simulink model "Shanthan_Heeirthan_EE469S3D_R45 (1)"  (R2023a)
settings: Solver=FixedStepDiscrete  StartTime=0.0  StopTime=120  FixedStep=dt0  RelTol=1e-3  EnableMultiTasking=on
PostLoadFcn:
  | %Set the size for the model
  | set_param(gcs,'Location',[10 10 1270 970])
  | %Set the zoom factor for the model
  | set_param(gcs,'ZoomFactor','100')
InitFcn:
  | tic
  | % Students Add call to their M-file HERE
  | Shanthan_Heeirthan_EE460_Final
  | INIT_S3D_01
StartFcn:
  | tend0=toc;
  | tic;
StopFcn:
  | tend=toc;
  | disp(['Simulation time = ' num2str(tout(end)) ' sec'])
  | disp(['Real time = ' num2str(tend) ' sec'])
  | title('DONE')
  | SCORE=round((max(0,120-tout(end)-tend0))*4+10*(40-FuelBurned)+sum(100*double(PDONE)-100*double(PDONE<.5)));
  | PlotS3D(PlotInput);
  | text(15,22,['S: ' num2str(SCORE)]);
values from neighbouring files (symbols this model uses):
  A = [0 1 0 0 0 0 ... (first row only)    [Shanthan_Heeirthan_EE460_Final (1).m]
  B = [0 0 0 ... (first row only)    [Shanthan_Heeirthan_EE460_Final (1).m]
  bm = [1 1 -1 -1 0 0 0 0; 0 0 0 0 -1 1 1 -1; -1 1 -1 1 3 -3 3 -3]    [Shanthan_Heeirthan_EE460_Final (1).m]
  C = [1 0 0 0 0 0 ... (first row only)    [Shanthan_Heeirthan_EE460_Final (1).m]
  D = [0 0 0 ... (first row only)    [Shanthan_Heeirthan_EE460_Final (1).m]
  Denchptheta = TFchptheta.Den{1}    [Shanthan_Heeirthan_EE460_Final (1).m]
  Denchpxy = TFchpxy.Den{1}    [Shanthan_Heeirthan_EE460_Final (1).m]
  Denclptheta = TFclptheta.Den{1}    [Shanthan_Heeirthan_EE460_Final (1).m]
  Denclpxy = TFclpxy.Den{1}    [Shanthan_Heeirthan_EE460_Final (1).m]
  Denlp = TFlp.Den{1}    [Shanthan_Heeirthan_EE460_Final (1).m]
  Kd = 2.1+0    (= 2.1)    [Shanthan_Heeirthan_EE460_Final (1).m]
  Ki = 0.0001    [Shanthan_Heeirthan_EE460_Final (1).m]
  Kp = 1.1+0.2    (= 1.3)    [Shanthan_Heeirthan_EE460_Final (1).m]
  L = place(A',C',ep)'    [Shanthan_Heeirthan_EE460_Final (1).m]
  Numchptheta = TFchptheta.Num{1}    [Shanthan_Heeirthan_EE460_Final (1).m]
  Numchpxy = TFchpxy.Num{1}    [Shanthan_Heeirthan_EE460_Final (1).m]
  Numclptheta = TFclptheta.Num{1}    [Shanthan_Heeirthan_EE460_Final (1).m]
  Numclpxy = TFclpxy.Num{1}    [Shanthan_Heeirthan_EE460_Final (1).m]
  Numlp = TFlp.Num{1}    [Shanthan_Heeirthan_EE460_Final (1).m]
  Pnewdata = [LVL.P1 LVL.P2 LVL.P3 LVL.P4]    [Shanthan_Heeirthan_EE460_Final (1).m]
  Sconfig = 1    [Shanthan_Heeirthan_EE460_Final (1).m]
  TFP1 = 2    [Shanthan_Heeirthan_EE460_Final (1).m]
  TFP1z = 1    [Shanthan_Heeirthan_EE460_Final (1).m]
  TFP2 = 2    [Shanthan_Heeirthan_EE460_Final (1).m]
  TFP2z = 1    [Shanthan_Heeirthan_EE460_Final (1).m]
  TFP3 = 2    [Shanthan_Heeirthan_EE460_Final (1).m]
  TFP3z = 1    [Shanthan_Heeirthan_EE460_Final (1).m]
  TFP4 = 2    [Shanthan_Heeirthan_EE460_Final (1).m]
  TFP4z = 1    [Shanthan_Heeirthan_EE460_Final (1).m]
  wcf = 2    [Shanthan_Heeirthan_EE460_Final (1).m]
  wcft = 10    [Shanthan_Heeirthan_EE460_Final (1).m]
undefined symbols (not defined in the file or in its folder): d2r, DiscIntNeverNeededParam, dt, dt0, fr, HM_S, HM_U, J, Jbase, JC0, L13, L24, LVL, M, M1, M2, M3, M4, mdti, Pdata, PTvec, r2d, SLIM, SQ, SSF, TOLdata, ULIM
libraries: simulink x85, aerolibanimutils x1, matrix_library x1
(part 6 of 7)

== system Shanthan_Heeirthan_EE469S3D_R45 (1)/control_law/CMD/CMDprocess/CommandTypes/Ramp1 ==
  ICCMDs : Inport
  Action Port : ActionPort  ActionPortLabel=if(u1 < 1.5)
  Bus Creator : BusCreator  Inputs=2
  Bus Selector : BusSelector  OutputSignals=X_CMD,Y_CMD
  Bus Selector1 : BusSelector  OutputSignals=CMDS.XdesCMD,CMDS.YdesCMD  OutputAsBus=on
  Gain : Gain
  Gain1 : Gain
  Gain2 : Gain
  Mux : Mux  Inputs=3
  Xcmd1 : Subsystem
  Ycmd : Subsystem
  Zcmd : Subsystem
  RMP_CMDS : Outport
  wires:
  Zcmd/1(ZCMD) -> Gain2/1
  Xcmd1/1(XCMD) -> Bus Creator/1
  Ycmd/1(XCMD) -> Bus Creator/2
  Mux/1 -> RMP_CMDS/1  "RMP_CMDS"
  Bus Creator/1 -> Bus Selector/1
  Bus Selector/2 -> Gain1/1  "<Y_CMD>"
  Bus Selector/1 -> Gain/1  "<X_CMD>"
  Gain/1 -> Mux/1
  Gain1/1 -> Mux/2
  ICCMDs/1 -> Bus Selector1/1, Zcmd/1(Sensed), Ycmd/1(ICCMDs), Xcmd1/1(ICCMDst)
  Bus Selector1/1 -> Zcmd/2(CMDS)  "CMDS"
  Gain2/1 -> Mux/3

== system Shanthan_Heeirthan_EE469S3D_R45 (1)/control_law/CMD/CMDprocess/CommandTypes/Ramp2 ==
  ICCMDs : Inport
  Action Port : ActionPort  ActionPortLabel=elseif( u1<3.5)
  Bus Creator : BusCreator  Inputs=2
  Bus Selector : BusSelector  OutputSignals=X_CMD,Y_CMD
  Bus Selector1 : BusSelector  OutputSignals=CMDS.XdesCMD,CMDS.YdesCMD  OutputAsBus=on
  Gain : Gain
  Gain1 : Gain
  Gain2 : Gain
  Mux : Mux  Inputs=3
  Xcmd1 : Subsystem
  Ycmd : Subsystem
  Zcmd : Subsystem
  RMP_CMDS : Outport
  wires:
  Zcmd/1(ZCMD) -> Gain2/1
  Xcmd1/1(XCMD) -> Bus Creator/1
  Ycmd/1(XCMD) -> Bus Creator/2
  Mux/1 -> RMP_CMDS/1  "RMP_CMDS"
  Bus Creator/1 -> Bus Selector/1
  Bus Selector/2 -> Gain1/1  "<Y_CMD>"
  Bus Selector/1 -> Gain/1  "<X_CMD>"
  Gain/1 -> Mux/1
  Gain1/1 -> Mux/2
  ICCMDs/1 -> Bus Selector1/1, Zcmd/1(Sensed), Ycmd/1(ICCMDs), Xcmd1/1(ICCMDst)
  Bus Selector1/1 -> Zcmd/2(CMDS)  "CMDS"
  Gain2/1 -> Mux/3

== system Shanthan_Heeirthan_EE469S3D_R45 (1)/control_law/CMD/CMDprocess/CommandTypes/Ramp3 ==
  ICCMDs : Inport
  Action Port : ActionPort  ActionPortLabel=else
  Bus Creator : BusCreator  Inputs=2
  Bus Selector : BusSelector  OutputSignals=X_CMD,Y_CMD
  Bus Selector1 : BusSelector  OutputSignals=CMDS.XdesCMD,CMDS.YdesCMD  OutputAsBus=on
  Gain : Gain
  Gain1 : Gain
  Gain2 : Gain
  Mux : Mux  Inputs=3
  Xcmd1 : Subsystem
  Ycmd : Subsystem
  Zcmd : Subsystem
  RMP_CMDS : Outport
  wires:
  Zcmd/1(ZCMD) -> Gain2/1
  Xcmd1/1(XCMD) -> Bus Creator/1
  Ycmd/1(XCMD) -> Bus Creator/2
  Mux/1 -> RMP_CMDS/1  "RMP_CMDS"
  Bus Creator/1 -> Bus Selector/1
  Bus Selector/2 -> Gain1/1  "<Y_CMD>"
  Bus Selector/1 -> Gain/1  "<X_CMD>"
  Gain/1 -> Mux/1
  Gain1/1 -> Mux/2
  ICCMDs/1 -> Bus Selector1/1, Zcmd/1(Sensed), Ycmd/1(ICCMDs), Xcmd1/1(ICCMDst)
  Bus Selector1/1 -> Zcmd/2(CMDS)  "CMDS"
  Gain2/1 -> Mux/3

== system Shanthan_Heeirthan_EE469S3D_R45 (1)/control_law/CMD/CMDprocess/CommandTypes/Ramp4 ==
  ICCMDs : Inport
  Action Port : ActionPort  ActionPortLabel=elseif(u1<2.5)
  Bus Creator : BusCreator  Inputs=2
  Bus Selector : BusSelector  OutputSignals=X_CMD,Y_CMD
  Bus Selector1 : BusSelector  OutputSignals=CMDS.XdesCMD,CMDS.YdesCMD  OutputAsBus=on
  Gain : Gain
  Gain1 : Gain
  Gain2 : Gain
  Mux : Mux  Inputs=3
  Xcmd1 : Subsystem
  Ycmd : Subsystem
  Zcmd : Subsystem
  RMP_CMDS : Outport
  wires:
  Zcmd/1(ZCMD) -> Gain2/1
  Xcmd1/1(XCMD) -> Bus Creator/1
  Ycmd/1(YCMD) -> Bus Creator/2
  Mux/1 -> RMP_CMDS/1  "RMP_CMDS"
  Bus Creator/1 -> Bus Selector/1
  Bus Selector/2 -> Gain1/1  "<Y_CMD>"
  Bus Selector/1 -> Gain/1  "<X_CMD>"
  Gain/1 -> Mux/1
  Gain1/1 -> Mux/2
  ICCMDs/1 -> Bus Selector1/1, Zcmd/1(Sensed), Ycmd/1(ICCMDs), Xcmd1/1(ICCMDst)
  Bus Selector1/1 -> Zcmd/2(CMDS)  "CMDS"
  Gain2/1 -> Mux/3

== system Shanthan_Heeirthan_EE469S3D_R45 (1)/control_law/CMD/CMDprocess/CommandTypes/Ramp1/Xcmd1 ==
  ICCMDst : Inport
  Bus Selector : BusSelector  OutputSignals=ICs.ICX,CMDS.XdesCMD
  Constant : Constant  Value=TFP1
  Gain : Gain  Gain=1/TFP1
  Gain1 : Gain
  Product : Product
  Sum : Sum  Inputs=|++
  Sum1 : Sum  Inputs=|-+
  VariableTimer : Subsystem
  XCMD : Outport
  wires:
  Gain1/1 -> XCMD/1  "X_CMD"
  Sum/1 -> Gain1/1  "qc"
  Bus Selector/2 -> Sum1/2  "<XdesCMD>"
  Bus Selector/1 -> Sum/1, Sum1/1  "<ICX>"
  ICCMDst/1 -> Bus Selector/1
  Constant/1 -> VariableTimer/1(TFramp)  "TFRamp"
  Product/1 -> Sum/2  "qcdot"
  Sum1/1 -> Gain/1
  VariableTimer/1(Time_sec) -> Product/2
  Gain/1 -> Product/1

== system Shanthan_Heeirthan_EE469S3D_R45 (1)/control_law/CMD/CMDprocess/CommandTypes/Ramp1/Ycmd ==
  ICCMDs : Inport
  Bus Selector : BusSelector  OutputSignals=ICs.ICY,CMDS.YdesCMD
  Constant : Constant  Value=TFP1
  Gain : Gain  Gain=1/TFP1
  Gain1 : Gain
  Product : Product
  Sum : Sum  Inputs=|++
  Sum1 : Sum  Inputs=|-+
  VariableTimer : Subsystem
  XCMD : Outport
  wires:
  VariableTimer/1(Time_sec) -> Product/2
  Product/1 -> Sum/2  "qcdot"
  Bus Selector/1 -> Sum/1, Sum1/1  "<ICY>"
  Gain1/1 -> XCMD/1  "Y_CMD"
  Sum/1 -> Gain1/1  "qc"
  Sum1/1 -> Gain/1
  Constant/1 -> VariableTimer/1(TFramp)  "TFRamp"
  ICCMDs/1 -> Bus Selector/1
  Bus Selector/2 -> Sum1/2  "<YdesCMD>"
  Gain/1 -> Product/1

== system Shanthan_Heeirthan_EE469S3D_R45 (1)/control_law/CMD/CMDprocess/CommandTypes/Ramp1/Zcmd ==
  Sensed : Inport
  CMDS : Inport  Port=2
  Bus Selector : BusSelector  OutputSignals=ICs.ICZ,CMDS.ZdesCMD
  Bus Selector2 : BusSelector  OutputSignals=Sensed.X1_m,Sensed.Y_m  OutputAsBus=on
  Constant : Constant  Value=0
  Data Type Conversion1 : DataTypeConversion  OutDataTypeStr=boolean  SaturateOnIntegerOverflow=off  RndMeth=Floor
  Gain : Gain  Gain=1/TFP1z
  If : If  IfExpression=u1 == 0
  Merge : Merge
  Product : Product
  StartTimer : Subsystem  TreatAsAtomicUnit=on
  Subsystem : Subsystem
  Sum : Sum  Inputs=|++
  Sum1 : Sum  Inputs=|-+
  Switch : Switch  Criteria=u2 > Threshold  SaturateOnIntegerOverflow=off  InputSameDT=off
  Terminator : Terminator
  ZCMD : Outport
  wires:
  Sum/1 -> ZCMD/1  "qc"
  Bus Selector/2 -> Sum1/2  "<ZdesCMD>"
  Gain/1 -> Product/1
  Bus Selector/1 -> Sum/1, Sum1/1  "<ICZ>"
  Sensed/1 -> Bus Selector2/1, Bus Selector/1
  Product/1 -> Sum/2  "qcdot"
  Sum1/1 -> Gain/1
  Switch/1 -> Product/2
  StartTimer/1(Out1) -> Switch/3
  Merge/1 -> Data Type Conversion1/1
  Data Type Conversion1/1 -> Switch/2, If/1
  Subsystem/1(Iftrue) -> Switch/1
  Subsystem/3(Toggle2) -> Merge/2
  CMDS/1 -> Subsystem/2(CMDS)  "CMDS"
  If/1 -> StartTimer/Action
  Bus Selector2/1 -> Subsystem/1(Sensed)  "Sensed"
  Subsystem/2(Toggle1) -> Merge/1
  Constant/1 -> Subsystem/3(Pmodeinit)  "Pmodeinit"
  If/2 -> Terminator/1

== system Shanthan_Heeirthan_EE469S3D_R45 (1)/control_law/CMD/CMDprocess/CommandTypes/Ramp2/Xcmd1 ==
  ICCMDst : Inport
  Bus Selector : BusSelector  OutputSignals=ICs.ICX,CMDS.XdesCMD
  Constant : Constant  Value=TFP3
  Gain : Gain  Gain=1/TFP3
  Gain1 : Gain
  Product : Product
  Sum : Sum  Inputs=|++
  Sum1 : Sum  Inputs=|-+
  VariableTimer : Subsystem
  XCMD : Outport
  wires:
  Gain1/1 -> XCMD/1  "X_CMD"
  Sum/1 -> Gain1/1  "qc"
  Bus Selector/2 -> Sum1/2  "<XdesCMD>"
  Bus Selector/1 -> Sum/1, Sum1/1  "<ICX>"
  ICCMDst/1 -> Bus Selector/1
  Constant/1 -> VariableTimer/1(TFramp)  "TFRamp"
  Product/1 -> Sum/2  "qcdot"
  Sum1/1 -> Gain/1
  VariableTimer/1(Time_sec) -> Product/2
  Gain/1 -> Product/1

== system Shanthan_Heeirthan_EE469S3D_R45 (1)/control_law/CMD/CMDprocess/CommandTypes/Ramp2/Ycmd ==
  ICCMDs : Inport
  Bus Selector : BusSelector  OutputSignals=ICs.ICY,CMDS.YdesCMD
  Constant : Constant  Value=TFP3
  Gain : Gain  Gain=1/TFP3
  Gain1 : Gain
  Product : Product
  Sum : Sum  Inputs=|++
  Sum1 : Sum  Inputs=|-+
  VariableTimer : Subsystem
  XCMD : Outport
  wires:
  VariableTimer/1(Time_sec) -> Product/2
  Product/1 -> Sum/2  "qcdot"
  Bus Selector/1 -> Sum/1, Sum1/1  "<ICY>"
  Gain1/1 -> XCMD/1  "Y_CMD"
  Sum/1 -> Gain1/1  "qc"
  Sum1/1 -> Gain/1
  Constant/1 -> VariableTimer/1(TFramp)  "TFRamp"
  ICCMDs/1 -> Bus Selector/1
  Bus Selector/2 -> Sum1/2  "<YdesCMD>"
  Gain/1 -> Product/1

== system Shanthan_Heeirthan_EE469S3D_R45 (1)/control_law/CMD/CMDprocess/CommandTypes/Ramp2/Zcmd ==
  Sensed : Inport
  CMDS : Inport  Port=2
  Bus Selector : BusSelector  OutputSignals=ICs.ICZ,CMDS.ZdesCMD
  Bus Selector2 : BusSelector  OutputSignals=Sensed.X1_m,Sensed.Y_m  OutputAsBus=on
  Constant : Constant  Value=0
  Data Type Conversion1 : DataTypeConversion  OutDataTypeStr=boolean  SaturateOnIntegerOverflow=off  RndMeth=Floor
  Gain : Gain  Gain=1/TFP3z
  If : If  IfExpression=u1 == 0
  Merge : Merge
  Product : Product
  StartTimer : Subsystem  TreatAsAtomicUnit=on
  Subsystem : Subsystem
  Sum : Sum  Inputs=|++
  Sum1 : Sum  Inputs=|-+
  Switch : Switch  Criteria=u2 > Threshold  SaturateOnIntegerOverflow=off  InputSameDT=off
  Terminator : Terminator
  ZCMD : Outport
  wires:
  Sum/1 -> ZCMD/1  "qc"
  Bus Selector/2 -> Sum1/2  "<ZdesCMD>"
  Gain/1 -> Product/1
  Bus Selector/1 -> Sum/1, Sum1/1  "<ICZ>"
  Sensed/1 -> Bus Selector2/1, Bus Selector/1
  Product/1 -> Sum/2  "qcdot"
  Sum1/1 -> Gain/1
  Switch/1 -> Product/2
  StartTimer/1(Out1) -> Switch/3
  Merge/1 -> Data Type Conversion1/1
  Data Type Conversion1/1 -> Switch/2, If/1
  Subsystem/1(Iftrue) -> Switch/1
  Subsystem/3(Toggle2) -> Merge/2
  CMDS/1 -> Subsystem/2(CMDS)  "CMDS"
  If/1 -> StartTimer/Action
  Bus Selector2/1 -> Subsystem/1(Sensed)  "Sensed"
  Subsystem/2(Toggle1) -> Merge/1
  Constant/1 -> Subsystem/3(Pmodeinit)  "Pmodeinit"
  If/2 -> Terminator/1

== system Shanthan_Heeirthan_EE469S3D_R45 (1)/control_law/CMD/CMDprocess/CommandTypes/Ramp3/Xcmd1 ==
  ICCMDst : Inport
  Bus Selector : BusSelector  OutputSignals=ICs.ICX,CMDS.XdesCMD
  Constant : Constant  Value=TFP4
  Gain : Gain  Gain=1/TFP4
  Gain1 : Gain
  Product : Product
  Sum : Sum  Inputs=|++
  Sum1 : Sum  Inputs=|-+
  VariableTimer : Subsystem
  XCMD : Outport
  wires:
  Gain1/1 -> XCMD/1  "X_CMD"
  Sum/1 -> Gain1/1  "qc"
  Bus Selector/2 -> Sum1/2  "<XdesCMD>"
  Bus Selector/1 -> Sum/1, Sum1/1  "<ICX>"
  ICCMDst/1 -> Bus Selector/1
  Constant/1 -> VariableTimer/1(TFramp)  "TFRamp"
  Product/1 -> Sum/2  "qcdot"
  Sum1/1 -> Gain/1
  VariableTimer/1(Time_sec) -> Product/2
  Gain/1 -> Product/1

== system Shanthan_Heeirthan_EE469S3D_R45 (1)/control_law/CMD/CMDprocess/CommandTypes/Ramp3/Ycmd ==
  ICCMDs : Inport
  Bus Selector : BusSelector  OutputSignals=ICs.ICY,CMDS.YdesCMD
  Constant : Constant  Value=TFP4
  Gain : Gain  Gain=1/TFP4
  Gain1 : Gain
  Product : Product
  Sum : Sum  Inputs=|++
  Sum1 : Sum  Inputs=|-+
  VariableTimer : Subsystem
  XCMD : Outport
  wires:
  VariableTimer/1(Time_sec) -> Product/2
  Product/1 -> Sum/2  "qcdot"
  Bus Selector/1 -> Sum/1, Sum1/1  "<ICY>"
  Gain1/1 -> XCMD/1  "Y_CMD"
  Sum/1 -> Gain1/1  "qc"
  Sum1/1 -> Gain/1
  Constant/1 -> VariableTimer/1(TFramp)  "TFRamp"
  ICCMDs/1 -> Bus Selector/1
  Bus Selector/2 -> Sum1/2  "<YdesCMD>"
  Gain/1 -> Product/1

== system Shanthan_Heeirthan_EE469S3D_R45 (1)/control_law/CMD/CMDprocess/CommandTypes/Ramp3/Zcmd ==
  Sensed : Inport
  CMDS : Inport  Port=2
  Bus Selector : BusSelector  OutputSignals=ICs.ICZ,CMDS.ZdesCMD
  Bus Selector2 : BusSelector  OutputSignals=Sensed.X1_m,Sensed.Y_m  OutputAsBus=on
  Constant : Constant  Value=0
  Data Type Conversion1 : DataTypeConversion  OutDataTypeStr=boolean  SaturateOnIntegerOverflow=off  RndMeth=Floor
  Gain : Gain  Gain=1/TFP4z
  If : If  IfExpression=u1 == 0
  Merge : Merge
  Product : Product
  StartTimer : Subsystem  TreatAsAtomicUnit=on
  Subsystem : Subsystem
  Sum : Sum  Inputs=|++
  Sum1 : Sum  Inputs=|-+
  Switch : Switch  Criteria=u2 > Threshold  SaturateOnIntegerOverflow=off  InputSameDT=off
  Terminator : Terminator
  ZCMD : Outport
  wires:
  Sum/1 -> ZCMD/1  "qc"
  Bus Selector/2 -> Sum1/2  "<ZdesCMD>"
  Gain/1 -> Product/1
  Bus Selector/1 -> Sum/1, Sum1/1  "<ICZ>"
  Sensed/1 -> Bus Selector2/1, Bus Selector/1
  Product/1 -> Sum/2  "qcdot"
  Sum1/1 -> Gain/1
  Switch/1 -> Product/2
  StartTimer/1(Out1) -> Switch/3
  Merge/1 -> Data Type Conversion1/1
  Data Type Conversion1/1 -> Switch/2, If/1
  Subsystem/1(Iftrue) -> Switch/1
  Subsystem/3(Toggle2) -> Merge/2
  CMDS/1 -> Subsystem/2(CMDS)  "CMDS"
  If/1 -> StartTimer/Action
  Bus Selector2/1 -> Subsystem/1(Sensed)  "Sensed"
  Subsystem/2(Toggle1) -> Merge/1
  Constant/1 -> Subsystem/3(Pmodeinit)  "Pmodeinit"
  If/2 -> Terminator/1

== system Shanthan_Heeirthan_EE469S3D_R45 (1)/control_law/CMD/CMDprocess/CommandTypes/Ramp4/Xcmd1 ==
  ICCMDst : Inport
  Bus Selector : BusSelector  OutputSignals=ICs.ICX,CMDS.XdesCMD
  Constant : Constant  Value=TFP2
  Gain : Gain  Gain=1/TFP2
  Gain1 : Gain
  Product : Product
  Sum : Sum  Inputs=|++
  Sum1 : Sum  Inputs=|-+
  VariableTimer : Subsystem
  XCMD : Outport
  wires:
  Gain1/1 -> XCMD/1  "X_CMD"
  Sum/1 -> Gain1/1  "qc"
  Bus Selector/2 -> Sum1/2  "<XdesCMD>"
  Bus Selector/1 -> Sum/1, Sum1/1  "<ICX>"
  ICCMDst/1 -> Bus Selector/1
  Constant/1 -> VariableTimer/1(TFramp)  "TFRamp"
  Product/1 -> Sum/2  "qcdot"
  Sum1/1 -> Gain/1
  VariableTimer/1(Time_sec) -> Product/2
  Gain/1 -> Product/1

== system Shanthan_Heeirthan_EE469S3D_R45 (1)/control_law/CMD/CMDprocess/CommandTypes/Ramp4/Ycmd ==
  ICCMDs : Inport
  Bus Selector : BusSelector  OutputSignals=ICs.ICY,CMDS.YdesCMD
  Constant : Constant  Value=TFP2
  Gain : Gain  Gain=1/TFP2
  Gain1 : Gain
  Product : Product
  Sum : Sum  Inputs=|++
  Sum1 : Sum  Inputs=|-+
  VariableTimer : Subsystem
  YCMD : Outport
  wires:
  VariableTimer/1(Time_sec) -> Product/2
  Product/1 -> Sum/2  "qcdot"
  Bus Selector/1 -> Sum/1, Sum1/1  "<ICY>"
  Gain1/1 -> YCMD/1  "Y_CMD"
  Sum/1 -> Gain1/1  "qc"
  Sum1/1 -> Gain/1
  Constant/1 -> VariableTimer/1(TFramp)  "TFRamp"
  ICCMDs/1 -> Bus Selector/1
  Bus Selector/2 -> Sum1/2  "<YdesCMD>"
  Gain/1 -> Product/1

== system Shanthan_Heeirthan_EE469S3D_R45 (1)/control_law/CMD/CMDprocess/CommandTypes/Ramp4/Zcmd ==
  Sensed : Inport
  CMDS : Inport  Port=2
  Bus Selector : BusSelector  OutputSignals=ICs.ICZ,CMDS.ZdesCMD
  Bus Selector2 : BusSelector  OutputSignals=Sensed.X1_m,Sensed.Y_m  OutputAsBus=on
  Constant : Constant  Value=0
  Data Type Conversion1 : DataTypeConversion  OutDataTypeStr=boolean  SaturateOnIntegerOverflow=off  RndMeth=Floor
  Gain : Gain  Gain=1/TFP2z
  If : If  IfExpression=u1 == 0
  Merge : Merge
  Product : Product
  StartTimer : Subsystem  TreatAsAtomicUnit=on
  Subsystem : Subsystem
  Sum : Sum  Inputs=|++
  Sum1 : Sum  Inputs=|-+
  Switch : Switch  Criteria=u2 > Threshold  SaturateOnIntegerOverflow=off  InputSameDT=off
  Terminator : Terminator
  ZCMD : Outport
  wires:
  Sum/1 -> ZCMD/1  "qc"
  Bus Selector/2 -> Sum1/2  "<ZdesCMD>"
  Gain/1 -> Product/1
  Bus Selector/1 -> Sum/1, Sum1/1  "<ICZ>"
  Sensed/1 -> Bus Selector/1, Bus Selector2/1
  Product/1 -> Sum/2  "qcdot"
  Sum1/1 -> Gain/1
  Switch/1 -> Product/2
  StartTimer/1(Out1) -> Switch/3
  Merge/1 -> Data Type Conversion1/1
  Data Type Conversion1/1 -> Switch/2, If/1
  Subsystem/1(Iftrue) -> Switch/1
  Subsystem/3(Toggle2) -> Merge/2
  CMDS/1 -> Subsystem/2(CMDS)  "CMDS"
  If/1 -> StartTimer/Action
  Bus Selector2/1 -> Subsystem/1(Sensed)  "Sensed"
  Subsystem/2(Toggle1) -> Merge/1
  Constant/1 -> Subsystem/3(Pmodeinit)  "Pmodeinit"
  If/2 -> Terminator/1

== system Shanthan_Heeirthan_EE469S3D_R45 (1)/control_law/CMD/CMDprocess/CommandTypes/Ramp1/Xcmd1/VariableTimer ==
  TFramp : Inport
  Constant : Constant  Value=dt
  DetectTFchange : Subsystem
  Logical Operator : Logic  Operator=OR  AllPortsSameDT=off  OutDataTypeStr=boolean
  Relational Operator : RelationalOperator  Operator=<=  OutDataTypeStr=boolean  RndMeth=Simplest  InputSameDT=off
  Sum : Sum  Inputs=|++
  Switch : Switch  Criteria=u2 > Threshold  SaturateOnIntegerOverflow=off  InputSameDT=off
  Unit Delay1 : UnitDelay  SampleTime=dt  HasFrameUpgradeWarning=on
  Unit Delay2 : UnitDelay  InitialCondition=-dt  SampleTime=dt  HasFrameUpgradeWarning=on
  Time_sec : Outport
  wires:
  Unit Delay2/1 -> Sum/2
  Sum/1 -> Relational Operator/2, Switch/3
  Constant/1 -> Sum/1
  Logical Operator/1 -> Switch/2
  Switch/1 -> Time_sec/1, Unit Delay1/1, Unit Delay2/1  "Time_sec"
  DetectTFchange/1(Out1) -> Switch/1
  Unit Delay1/1 -> DetectTFchange/1(In1)  "TimeZ_sec"
  DetectTFchange/2(Out2) -> Logical Operator/1
  TFramp/1 -> DetectTFchange/2(In3), Relational Operator/1
  Relational Operator/1 -> Logical Operator/2  "Reset1"

== system Shanthan_Heeirthan_EE469S3D_R45 (1)/control_law/CMD/CMDprocess/CommandTypes/Ramp1/Ycmd/VariableTimer ==
  TFramp : Inport
  Constant : Constant  Value=dt
  DetectTFchange : Subsystem
  Logical Operator : Logic  Operator=OR  AllPortsSameDT=off  OutDataTypeStr=boolean
  Relational Operator : RelationalOperator  Operator=<=  OutDataTypeStr=boolean  RndMeth=Simplest  InputSameDT=off
  Sum : Sum  Inputs=|++
  Switch : Switch  Criteria=u2 > Threshold  SaturateOnIntegerOverflow=off  InputSameDT=off
  Unit Delay1 : UnitDelay  SampleTime=dt  HasFrameUpgradeWarning=on
  Unit Delay2 : UnitDelay  InitialCondition=-dt  SampleTime=dt  HasFrameUpgradeWarning=on
  Time_sec : Outport
  wires:
  Unit Delay2/1 -> Sum/2
  Sum/1 -> Relational Operator/2, Switch/3
  Constant/1 -> Sum/1
  Logical Operator/1 -> Switch/2
  Switch/1 -> Time_sec/1, Unit Delay1/1, Unit Delay2/1  "Time_sec"
  DetectTFchange/1(Out1) -> Switch/1
  Unit Delay1/1 -> DetectTFchange/1(In1)  "TimeZ_sec"
  DetectTFchange/2(Out2) -> Logical Operator/1
  TFramp/1 -> DetectTFchange/2(In3), Relational Operator/1
  Relational Operator/1 -> Logical Operator/2  "Reset1"

== system Shanthan_Heeirthan_EE469S3D_R45 (1)/control_law/CMD/CMDprocess/CommandTypes/Ramp1/Zcmd/StartTimer ==
  Action Port : ActionPort  ActionPortLabel=if(u1 == 0)
  Constant : Constant  Value=TFP1z
  VariableTimer : Subsystem
  Out1 : Outport
  wires:
  Constant/1 -> VariableTimer/1(TFramp)  "TFRamp"
  VariableTimer/1(Time_sec) -> Out1/1

== system Shanthan_Heeirthan_EE469S3D_R45 (1)/control_law/CMD/CMDprocess/CommandTypes/Ramp1/Zcmd/Subsystem ==
  Sensed : Inport
  CMDS : Inport  Port=2
  Pmodeinit : Inport  Port=3
  Constant2 : Constant  Value=0
  False : Subsystem  TreatAsAtomicUnit=on
  If : If  IfExpression=u1 ==0
  If1 : If  IfExpression=u1 ==0
  Merge : Merge
  Mode1 : Subsystem  TreatAsAtomicUnit=on
  Mode2 : Subsystem  TreatAsAtomicUnit=on
  Saturation : Saturate  UpperLimit=1  LowerLimit=0
  Sum : Sum  Inputs=|++
  Threshold : Subsystem
  True : Subsystem  TreatAsAtomicUnit=on
  Unit Delay : UnitDelay  SampleTime=dt  HasFrameUpgradeWarning=on
  Iftrue : Outport
  Toggle1 : Outport  Port=2
  Toggle2 : Outport  Port=3
  wires:
  Constant2/1 -> Iftrue/1  "zero"
  If/2 -> False/Action
  If/1 -> True/Action
  Sensed/1 -> Threshold/2(CMDS)  "Sensed"
  CMDS/1 -> Threshold/1(Sensed)
  True/1(Out1) -> Toggle1/1
  Threshold/1(Threshold) -> If1/1
  Pmodeinit/1 -> Sum/1
  If1/1 -> Mode2/Action
  If1/2 -> Mode1/Action
  Mode2/1(Pmode1) -> Merge/1
  Mode1/1(Pmode1) -> Merge/2
  Merge/1 -> Unit Delay/1
  Saturation/1 -> If/1, Mode1/1(Pmode), Mode2/1(Pmode)  "Pmode"
  Unit Delay/1 -> Sum/2
  Sum/1 -> Saturation/1
  False/1(Out1) -> Toggle2/1

== system Shanthan_Heeirthan_EE469S3D_R45 (1)/control_law/CMD/CMDprocess/CommandTypes/Ramp2/Xcmd1/VariableTimer ==
  TFramp : Inport
  Constant : Constant  Value=dt
  DetectTFchange : Subsystem
  Logical Operator : Logic  Operator=OR  AllPortsSameDT=off  OutDataTypeStr=boolean
  Relational Operator : RelationalOperator  Operator=<=  OutDataTypeStr=boolean  RndMeth=Simplest  InputSameDT=off
  Sum : Sum  Inputs=|++
  Switch : Switch  Criteria=u2 > Threshold  SaturateOnIntegerOverflow=off  InputSameDT=off
  Unit Delay1 : UnitDelay  SampleTime=dt  HasFrameUpgradeWarning=on
  Unit Delay2 : UnitDelay  InitialCondition=-dt  SampleTime=dt  HasFrameUpgradeWarning=on
  Time_sec : Outport
  wires:
  Unit Delay2/1 -> Sum/2
  Sum/1 -> Relational Operator/2, Switch/3
  Constant/1 -> Sum/1
  Logical Operator/1 -> Switch/2
  Switch/1 -> Time_sec/1, Unit Delay1/1, Unit Delay2/1  "Time_sec"
  DetectTFchange/1(Out1) -> Switch/1
  Unit Delay1/1 -> DetectTFchange/1(In1)  "TimeZ_sec"
  DetectTFchange/2(Out2) -> Logical Operator/1
  TFramp/1 -> DetectTFchange/2(In3), Relational Operator/1
  Relational Operator/1 -> Logical Operator/2  "Reset1"

== system Shanthan_Heeirthan_EE469S3D_R45 (1)/control_law/CMD/CMDprocess/CommandTypes/Ramp2/Ycmd/VariableTimer ==
  TFramp : Inport
  Constant : Constant  Value=dt
  DetectTFchange : Subsystem
  Logical Operator : Logic  Operator=OR  AllPortsSameDT=off  OutDataTypeStr=boolean
  Relational Operator : RelationalOperator  Operator=<=  OutDataTypeStr=boolean  RndMeth=Simplest  InputSameDT=off
  Sum : Sum  Inputs=|++
  Switch : Switch  Criteria=u2 > Threshold  SaturateOnIntegerOverflow=off  InputSameDT=off
  Unit Delay1 : UnitDelay  SampleTime=dt  HasFrameUpgradeWarning=on
  Unit Delay2 : UnitDelay  InitialCondition=-dt  SampleTime=dt  HasFrameUpgradeWarning=on
  Time_sec : Outport
  wires:
  Unit Delay2/1 -> Sum/2
  Sum/1 -> Relational Operator/2, Switch/3
  Constant/1 -> Sum/1
  Logical Operator/1 -> Switch/2
  Switch/1 -> Time_sec/1, Unit Delay1/1, Unit Delay2/1  "Time_sec"
  DetectTFchange/1(Out1) -> Switch/1
  Unit Delay1/1 -> DetectTFchange/1(In1)  "TimeZ_sec"
  DetectTFchange/2(Out2) -> Logical Operator/1
  TFramp/1 -> DetectTFchange/2(In3), Relational Operator/1
  Relational Operator/1 -> Logical Operator/2  "Reset1"

== system Shanthan_Heeirthan_EE469S3D_R45 (1)/control_law/CMD/CMDprocess/CommandTypes/Ramp2/Zcmd/StartTimer ==
  Action Port : ActionPort  ActionPortLabel=if(u1 == 0)
  Constant : Constant  Value=TFP3z
  VariableTimer : Subsystem
  Out1 : Outport
  wires:
  Constant/1 -> VariableTimer/1(TFramp)  "TFRamp"
  VariableTimer/1(Time_sec) -> Out1/1

== system Shanthan_Heeirthan_EE469S3D_R45 (1)/control_law/CMD/CMDprocess/CommandTypes/Ramp2/Zcmd/Subsystem ==
  Sensed : Inport
  CMDS : Inport  Port=2
  Pmodeinit : Inport  Port=3
  Constant2 : Constant  Value=0
  False : Subsystem  TreatAsAtomicUnit=on
  If : If  IfExpression=u1 ==0
  If1 : If  IfExpression=u1 ==0
  Merge : Merge
  Mode1 : Subsystem  TreatAsAtomicUnit=on
  Mode2 : Subsystem  TreatAsAtomicUnit=on
  Saturation : Saturate  UpperLimit=1  LowerLimit=0
  Sum : Sum  Inputs=|++
  Threshold : Subsystem
  True : Subsystem  TreatAsAtomicUnit=on
  Unit Delay : UnitDelay  SampleTime=dt  HasFrameUpgradeWarning=on
  Iftrue : Outport
  Toggle1 : Outport  Port=2
  Toggle2 : Outport  Port=3
  wires:
  Constant2/1 -> Iftrue/1  "zero"
  If/2 -> False/Action
  If/1 -> True/Action
  Sensed/1 -> Threshold/2(CMDS)  "Sensed"
  CMDS/1 -> Threshold/1(Sensed)
  True/1(Out1) -> Toggle1/1
  Threshold/1(Threshold) -> If1/1
  Pmodeinit/1 -> Sum/1
  If1/1 -> Mode2/Action
  If1/2 -> Mode1/Action
  Mode2/1(Pmode1) -> Merge/1
  Mode1/1(Pmode1) -> Merge/2
  Merge/1 -> Unit Delay/1
  Saturation/1 -> Mode1/1(Pmode), Mode2/1(Pmode), If/1  "Pmode"
  Unit Delay/1 -> Sum/2
  Sum/1 -> Saturation/1
  False/1(Out1) -> Toggle2/1

== system Shanthan_Heeirthan_EE469S3D_R45 (1)/control_law/CMD/CMDprocess/CommandTypes/Ramp3/Xcmd1/VariableTimer ==
  TFramp : Inport
  Constant : Constant  Value=dt
  DetectTFchange : Subsystem
  Logical Operator : Logic  Operator=OR  AllPortsSameDT=off  OutDataTypeStr=boolean
  Relational Operator : RelationalOperator  Operator=<=  OutDataTypeStr=boolean  RndMeth=Simplest  InputSameDT=off
  Sum : Sum  Inputs=|++
  Switch : Switch  Criteria=u2 > Threshold  SaturateOnIntegerOverflow=off  InputSameDT=off
  Unit Delay1 : UnitDelay  SampleTime=dt  HasFrameUpgradeWarning=on
  Unit Delay2 : UnitDelay  InitialCondition=-dt  SampleTime=dt  HasFrameUpgradeWarning=on
  Time_sec : Outport
  wires:
  Unit Delay2/1 -> Sum/2
  Sum/1 -> Relational Operator/2, Switch/3
  Constant/1 -> Sum/1
  Logical Operator/1 -> Switch/2
  Switch/1 -> Time_sec/1, Unit Delay1/1, Unit Delay2/1  "Time_sec"
  DetectTFchange/1(Out1) -> Switch/1
  Unit Delay1/1 -> DetectTFchange/1(In1)  "TimeZ_sec"
  DetectTFchange/2(Out2) -> Logical Operator/1
  TFramp/1 -> DetectTFchange/2(In3), Relational Operator/1
  Relational Operator/1 -> Logical Operator/2  "Reset1"

== system Shanthan_Heeirthan_EE469S3D_R45 (1)/control_law/CMD/CMDprocess/CommandTypes/Ramp3/Ycmd/VariableTimer ==
  TFramp : Inport
  Constant : Constant  Value=dt
  DetectTFchange : Subsystem
  Logical Operator : Logic  Operator=OR  AllPortsSameDT=off  OutDataTypeStr=boolean
  Relational Operator : RelationalOperator  Operator=<=  OutDataTypeStr=boolean  RndMeth=Simplest  InputSameDT=off
  Sum : Sum  Inputs=|++
  Switch : Switch  Criteria=u2 > Threshold  SaturateOnIntegerOverflow=off  InputSameDT=off
  Unit Delay1 : UnitDelay  SampleTime=dt  HasFrameUpgradeWarning=on
  Unit Delay2 : UnitDelay  InitialCondition=-dt  SampleTime=dt  HasFrameUpgradeWarning=on
  Time_sec : Outport
  wires:
  Unit Delay2/1 -> Sum/2
  Sum/1 -> Relational Operator/2, Switch/3
  Constant/1 -> Sum/1
  Logical Operator/1 -> Switch/2
  Switch/1 -> Time_sec/1, Unit Delay1/1, Unit Delay2/1  "Time_sec"
  DetectTFchange/1(Out1) -> Switch/1
  Unit Delay1/1 -> DetectTFchange/1(In1)  "TimeZ_sec"
  DetectTFchange/2(Out2) -> Logical Operator/1
  TFramp/1 -> DetectTFchange/2(In3), Relational Operator/1
  Relational Operator/1 -> Logical Operator/2  "Reset1"

== system Shanthan_Heeirthan_EE469S3D_R45 (1)/control_law/CMD/CMDprocess/CommandTypes/Ramp3/Zcmd/StartTimer ==
  Action Port : ActionPort  ActionPortLabel=if(u1 == 0)
  Constant : Constant  Value=TFP4z
  VariableTimer : Subsystem
  Out1 : Outport
  wires:
  Constant/1 -> VariableTimer/1(TFramp)  "TFRamp"
  VariableTimer/1(Time_sec) -> Out1/1

== system Shanthan_Heeirthan_EE469S3D_R45 (1)/control_law/CMD/CMDprocess/CommandTypes/Ramp3/Zcmd/Subsystem ==
  Sensed : Inport
  CMDS : Inport  Port=2
  Pmodeinit : Inport  Port=3
  Constant2 : Constant  Value=0
  False : Subsystem  TreatAsAtomicUnit=on
  If : If  IfExpression=u1 ==0
  If1 : If  IfExpression=u1 ==0
  Merge : Merge
  Mode1 : Subsystem  TreatAsAtomicUnit=on
  Mode2 : Subsystem  TreatAsAtomicUnit=on
  Saturation : Saturate  UpperLimit=1  LowerLimit=0
  Sum : Sum  Inputs=|++
  Threshold : Subsystem
  True : Subsystem  TreatAsAtomicUnit=on
  Unit Delay : UnitDelay  SampleTime=dt  HasFrameUpgradeWarning=on
  Iftrue : Outport
  Toggle1 : Outport  Port=2
  Toggle2 : Outport  Port=3
  wires:
  Constant2/1 -> Iftrue/1  "zero"
  If/2 -> False/Action
  If/1 -> True/Action
  Sensed/1 -> Threshold/2(CMDS)  "Sensed"
  CMDS/1 -> Threshold/1(Sensed)
  True/1(Out1) -> Toggle1/1
  Threshold/1(Threshold) -> If1/1
  Pmodeinit/1 -> Sum/1
  If1/1 -> Mode2/Action
  If1/2 -> Mode1/Action
  Mode2/1(Pmode1) -> Merge/1
  Mode1/1(Pmode1) -> Merge/2
  Merge/1 -> Unit Delay/1
  Saturation/1 -> If/1, Mode1/1(Pmode), Mode2/1(Pmode)  "Pmode"
  Unit Delay/1 -> Sum/2
  Sum/1 -> Saturation/1
  False/1(Out1) -> Toggle2/1

== system Shanthan_Heeirthan_EE469S3D_R45 (1)/control_law/CMD/CMDprocess/CommandTypes/Ramp4/Xcmd1/VariableTimer ==
  TFramp : Inport
  Constant : Constant  Value=dt
  DetectTFchange : Subsystem
  Logical Operator : Logic  Operator=OR  AllPortsSameDT=off  OutDataTypeStr=boolean
  Relational Operator : RelationalOperator  Operator=<=  OutDataTypeStr=boolean  RndMeth=Simplest  InputSameDT=off
  Sum : Sum  Inputs=|++
  Switch : Switch  Criteria=u2 > Threshold  SaturateOnIntegerOverflow=off  InputSameDT=off
  Unit Delay1 : UnitDelay  SampleTime=dt  HasFrameUpgradeWarning=on
  Unit Delay2 : UnitDelay  InitialCondition=-dt  SampleTime=dt  HasFrameUpgradeWarning=on
  Time_sec : Outport
  wires:
  Unit Delay2/1 -> Sum/2
  Sum/1 -> Relational Operator/2, Switch/3
  Constant/1 -> Sum/1
  Logical Operator/1 -> Switch/2
  Switch/1 -> Time_sec/1, Unit Delay1/1, Unit Delay2/1  "Time_sec"
  DetectTFchange/1(Out1) -> Switch/1
  Unit Delay1/1 -> DetectTFchange/1(In1)  "TimeZ_sec"
  DetectTFchange/2(Out2) -> Logical Operator/1
  TFramp/1 -> DetectTFchange/2(In3), Relational Operator/1
  Relational Operator/1 -> Logical Operator/2  "Reset1"

== system Shanthan_Heeirthan_EE469S3D_R45 (1)/control_law/CMD/CMDprocess/CommandTypes/Ramp4/Ycmd/VariableTimer ==
  TFramp : Inport
  Constant : Constant  Value=dt
  DetectTFchange : Subsystem
  Logical Operator : Logic  Operator=OR  AllPortsSameDT=off  OutDataTypeStr=boolean
  Relational Operator : RelationalOperator  Operator=<=  OutDataTypeStr=boolean  RndMeth=Simplest  InputSameDT=off
  Sum : Sum  Inputs=|++
  Switch : Switch  Criteria=u2 > Threshold  SaturateOnIntegerOverflow=off  InputSameDT=off
  Unit Delay1 : UnitDelay  SampleTime=dt  HasFrameUpgradeWarning=on
  Unit Delay2 : UnitDelay  InitialCondition=-dt  SampleTime=dt  HasFrameUpgradeWarning=on
  Time_sec : Outport
  wires:
  Unit Delay2/1 -> Sum/2
  Sum/1 -> Relational Operator/2, Switch/3
  Constant/1 -> Sum/1
  Logical Operator/1 -> Switch/2
  Switch/1 -> Time_sec/1, Unit Delay1/1, Unit Delay2/1  "Time_sec"
  DetectTFchange/1(Out1) -> Switch/1
  Unit Delay1/1 -> DetectTFchange/1(In1)  "TimeZ_sec"
  DetectTFchange/2(Out2) -> Logical Operator/1
  TFramp/1 -> DetectTFchange/2(In3), Relational Operator/1
  Relational Operator/1 -> Logical Operator/2  "Reset1"

== system Shanthan_Heeirthan_EE469S3D_R45 (1)/control_law/CMD/CMDprocess/CommandTypes/Ramp4/Zcmd/StartTimer ==
  Action Port : ActionPort  ActionPortLabel=if(u1 == 0)
  Constant : Constant  Value=TFP2z
  VariableTimer : Subsystem
  Out1 : Outport
  wires:
  Constant/1 -> VariableTimer/1(TFramp)  "TFRamp"
  VariableTimer/1(Time_sec) -> Out1/1

== system Shanthan_Heeirthan_EE469S3D_R45 (1)/control_law/CMD/CMDprocess/CommandTypes/Ramp4/Zcmd/Subsystem ==
  Sensed : Inport
  CMDS : Inport  Port=2
  Pmodeinit : Inport  Port=3
  Constant2 : Constant  Value=0
  False : Subsystem  TreatAsAtomicUnit=on
  If : If  IfExpression=u1 ==0
  If1 : If  IfExpression=u1 ==0
  Merge : Merge
  Mode1 : Subsystem  TreatAsAtomicUnit=on
  Mode2 : Subsystem  TreatAsAtomicUnit=on
  Saturation : Saturate  UpperLimit=1  LowerLimit=0
  Sum : Sum  Inputs=|++
  Threshold : Subsystem
  True : Subsystem  TreatAsAtomicUnit=on
  Unit Delay : UnitDelay  SampleTime=dt  HasFrameUpgradeWarning=on
  Iftrue : Outport
  Toggle1 : Outport  Port=2
  Toggle2 : Outport  Port=3
  wires:
  Constant2/1 -> Iftrue/1  "zero"
  If/2 -> False/Action
  If/1 -> True/Action
  Sensed/1 -> Threshold/2(CMDS)  "Sensed"
  CMDS/1 -> Threshold/1(Sensed)
  True/1(Out1) -> Toggle1/1
  Threshold/1(Threshold) -> If1/1
  Pmodeinit/1 -> Sum/1
  If1/1 -> Mode2/Action
  If1/2 -> Mode1/Action
  Mode2/1(Pmode1) -> Merge/1
  Mode1/1(Pmode1) -> Merge/2
  Merge/1 -> Unit Delay/1
  Saturation/1 -> If/1, Mode1/1(Pmode), Mode2/1(Pmode)  "Pmode"
  Unit Delay/1 -> Sum/2
  Sum/1 -> Saturation/1
  False/1(Out1) -> Toggle2/1

== system Shanthan_Heeirthan_EE469S3D_R45 (1)/control_law/CMD/CMDprocess/CommandTypes/Ramp1/Xcmd1/VariableTimer/DetectTFchange ==
  In1 : Inport
  In3 : Inport  Port=2
  Constant : Constant  Value=0
  Relational Operator1 : RelationalOperator  Operator=~=  OutDataTypeStr=boolean  RndMeth=Simplest  InputSameDT=off
  Switch3 : Switch  Criteria=u2 > Threshold  SaturateOnIntegerOverflow=off  InputSameDT=off
  Unit Delay : UnitDelay  InitialCondition=-dt  SampleTime=dt  HasFrameUpgradeWarning=on
  Out1 : Outport
  Out2 : Outport  Port=2
  wires:
  Switch3/1 -> Out1/1  "ResetValue"
  In3/1 -> Relational Operator1/1, Unit Delay/1
  Unit Delay/1 -> Relational Operator1/2
  Relational Operator1/1 -> Out2/1, Switch3/2  "Reset2"
  In1/1 -> Switch3/3
  Constant/1 -> Switch3/1

== system Shanthan_Heeirthan_EE469S3D_R45 (1)/control_law/CMD/CMDprocess/CommandTypes/Ramp1/Ycmd/VariableTimer/DetectTFchange ==
  In1 : Inport
  In3 : Inport  Port=2
  Constant : Constant  Value=0
  Relational Operator1 : RelationalOperator  Operator=~=  OutDataTypeStr=boolean  RndMeth=Simplest  InputSameDT=off
  Switch3 : Switch  Criteria=u2 > Threshold  SaturateOnIntegerOverflow=off  InputSameDT=off
  Unit Delay : UnitDelay  InitialCondition=-dt  SampleTime=dt  HasFrameUpgradeWarning=on
  Out1 : Outport
  Out2 : Outport  Port=2
  wires:
  Switch3/1 -> Out1/1  "ResetValue"
  In3/1 -> Relational Operator1/1, Unit Delay/1
  Unit Delay/1 -> Relational Operator1/2
  Relational Operator1/1 -> Out2/1, Switch3/2  "Reset2"
  In1/1 -> Switch3/3
  Constant/1 -> Switch3/1

== system Shanthan_Heeirthan_EE469S3D_R45 (1)/control_law/CMD/CMDprocess/CommandTypes/Ramp1/Zcmd/StartTimer/VariableTimer ==
  TFramp : Inport
  Constant : Constant  Value=dt
  DetectTFchange : Subsystem
  Logical Operator : Logic  Operator=OR  AllPortsSameDT=off  OutDataTypeStr=boolean
  Relational Operator : RelationalOperator  Operator=<=  OutDataTypeStr=boolean  RndMeth=Simplest  InputSameDT=off
  Sum : Sum  Inputs=|++
  Switch : Switch  Criteria=u2 > Threshold  SaturateOnIntegerOverflow=off  InputSameDT=off
  Unit Delay1 : UnitDelay  SampleTime=dt  HasFrameUpgradeWarning=on
  Unit Delay2 : UnitDelay  InitialCondition=-dt  SampleTime=dt  HasFrameUpgradeWarning=on
  Time_sec : Outport
  wires:
  Unit Delay2/1 -> Sum/2
  Sum/1 -> Relational Operator/2, Switch/3
  Constant/1 -> Sum/1
  Logical Operator/1 -> Switch/2
  Switch/1 -> Time_sec/1, Unit Delay1/1, Unit Delay2/1  "Time_sec"
  DetectTFchange/1(Out1) -> Switch/1
  Unit Delay1/1 -> DetectTFchange/1(In1)  "TimeZ_sec"
  DetectTFchange/2(Out2) -> Logical Operator/1
  TFramp/1 -> DetectTFchange/2(In3), Relational Operator/1
  Relational Operator/1 -> Logical Operator/2  "Reset1"

== system Shanthan_Heeirthan_EE469S3D_R45 (1)/control_law/CMD/CMDprocess/CommandTypes/Ramp1/Zcmd/Subsystem/False ==
  Action Port : ActionPort  ActionPortLabel=else
  Constant : Constant  Value=0
  Out1 : Outport
  wires:
  Constant/1 -> Out1/1  "zero"

== system Shanthan_Heeirthan_EE469S3D_R45 (1)/control_law/CMD/CMDprocess/CommandTypes/Ramp1/Zcmd/Subsystem/Mode1 ==
  Pmode : Inport
  Action Port : ActionPort  ActionPortLabel=else
  Pmode1 : Outport
  wires:
  Pmode/1 -> Pmode1/1

== system Shanthan_Heeirthan_EE469S3D_R45 (1)/control_law/CMD/CMDprocess/CommandTypes/Ramp1/Zcmd/Subsystem/Mode2 ==
  Pmode : Inport
  Action Port : ActionPort  ActionPortLabel=if(u1 ==0)
  Constant : Constant
  Sum : Sum  Inputs=|++
  Pmode1 : Outport
  wires:
  Pmode/1 -> Sum/1
  Constant/1 -> Sum/2
  Sum/1 -> Pmode1/1  "Pmode"

== system Shanthan_Heeirthan_EE469S3D_R45 (1)/control_law/CMD/CMDprocess/CommandTypes/Ramp1/Zcmd/Subsystem/Threshold ==
  Sensed : Inport
  CMDS : Inport  Port=2
  Abs : Abs  SaturateOnIntegerOverflow=off
  Bus to Vector : BusToVector
  Bus to Vector1 : BusToVector
  Constant1 : Constant  Value=[TOLdata(1,1);TOLdata(2,1)]
  Data Type Conversion : DataTypeConversion  OutDataTypeStr=double  SaturateOnIntegerOverflow=off  RndMeth=Floor
  Relational Operator : RelationalOperator  OutDataTypeStr=boolean  RndMeth=Simplest  InputSameDT=off
  Sum2 : Sum  Inputs=|+-
  Sum3 : Sum  Inputs=+
  Threshold : Outport
  wires:
  Sum2/1 -> Abs/1
  Bus to Vector/1 -> Sum2/1
  Bus to Vector1/1 -> Sum2/2
  Constant1/1 -> Relational Operator/2
  Abs/1 -> Relational Operator/1
  Data Type Conversion/1 -> Sum3/1
  Sensed/1 -> Bus to Vector1/1
  Relational Operator/1 -> Data Type Conversion/1
  CMDS/1 -> Bus to Vector/1
  Sum3/1 -> Threshold/1  "threshold"

== system Shanthan_Heeirthan_EE469S3D_R45 (1)/control_law/CMD/CMDprocess/CommandTypes/Ramp1/Zcmd/Subsystem/True ==
  Action Port : ActionPort  ActionPortLabel=if(u1 ==0)
  Constant : Constant
  Out1 : Outport
  wires:
  Constant/1 -> Out1/1  "one"

== system Shanthan_Heeirthan_EE469S3D_R45 (1)/control_law/CMD/CMDprocess/CommandTypes/Ramp2/Xcmd1/VariableTimer/DetectTFchange ==
  In1 : Inport
  In3 : Inport  Port=2
  Constant : Constant  Value=0
  Relational Operator1 : RelationalOperator  Operator=~=  OutDataTypeStr=boolean  RndMeth=Simplest  InputSameDT=off
  Switch3 : Switch  Criteria=u2 > Threshold  SaturateOnIntegerOverflow=off  InputSameDT=off
  Unit Delay : UnitDelay  InitialCondition=-dt  SampleTime=dt  HasFrameUpgradeWarning=on
  Out1 : Outport
  Out2 : Outport  Port=2
  wires:
  Switch3/1 -> Out1/1  "ResetValue"
  In3/1 -> Relational Operator1/1, Unit Delay/1
  Unit Delay/1 -> Relational Operator1/2
  Relational Operator1/1 -> Out2/1, Switch3/2  "Reset2"
  In1/1 -> Switch3/3
  Constant/1 -> Switch3/1

== system Shanthan_Heeirthan_EE469S3D_R45 (1)/control_law/CMD/CMDprocess/CommandTypes/Ramp2/Ycmd/VariableTimer/DetectTFchange ==
  In1 : Inport
  In3 : Inport  Port=2
  Constant : Constant  Value=0
  Relational Operator1 : RelationalOperator  Operator=~=  OutDataTypeStr=boolean  RndMeth=Simplest  InputSameDT=off
  Switch3 : Switch  Criteria=u2 > Threshold  SaturateOnIntegerOverflow=off  InputSameDT=off
  Unit Delay : UnitDelay  InitialCondition=-dt  SampleTime=dt  HasFrameUpgradeWarning=on
  Out1 : Outport
  Out2 : Outport  Port=2
  wires:
  Switch3/1 -> Out1/1  "ResetValue"
  In3/1 -> Relational Operator1/1, Unit Delay/1
  Unit Delay/1 -> Relational Operator1/2
  Relational Operator1/1 -> Out2/1, Switch3/2  "Reset2"
  In1/1 -> Switch3/3
  Constant/1 -> Switch3/1

== system Shanthan_Heeirthan_EE469S3D_R45 (1)/control_law/CMD/CMDprocess/CommandTypes/Ramp2/Zcmd/StartTimer/VariableTimer ==
  TFramp : Inport
  Constant : Constant  Value=dt
  DetectTFchange : Subsystem
  Logical Operator : Logic  Operator=OR  AllPortsSameDT=off  OutDataTypeStr=boolean
  Relational Operator : RelationalOperator  Operator=<=  OutDataTypeStr=boolean  RndMeth=Simplest  InputSameDT=off
  Sum : Sum  Inputs=|++
  Switch : Switch  Criteria=u2 > Threshold  SaturateOnIntegerOverflow=off  InputSameDT=off
  Unit Delay1 : UnitDelay  SampleTime=dt  HasFrameUpgradeWarning=on
  Unit Delay2 : UnitDelay  InitialCondition=-dt  SampleTime=dt  HasFrameUpgradeWarning=on
  Time_sec : Outport
  wires:
  Unit Delay2/1 -> Sum/2
  Sum/1 -> Relational Operator/2, Switch/3
  Constant/1 -> Sum/1
  Logical Operator/1 -> Switch/2
  Switch/1 -> Time_sec/1, Unit Delay1/1, Unit Delay2/1  "Time_sec"
  DetectTFchange/1(Out1) -> Switch/1
  Unit Delay1/1 -> DetectTFchange/1(In1)  "TimeZ_sec"
  DetectTFchange/2(Out2) -> Logical Operator/1
  TFramp/1 -> DetectTFchange/2(In3), Relational Operator/1
  Relational Operator/1 -> Logical Operator/2  "Reset1"

== system Shanthan_Heeirthan_EE469S3D_R45 (1)/control_law/CMD/CMDprocess/CommandTypes/Ramp2/Zcmd/Subsystem/False ==
  Action Port : ActionPort  ActionPortLabel=else
  Constant : Constant  Value=0
  Out1 : Outport
  wires:
  Constant/1 -> Out1/1  "zero"

== system Shanthan_Heeirthan_EE469S3D_R45 (1)/control_law/CMD/CMDprocess/CommandTypes/Ramp2/Zcmd/Subsystem/Mode1 ==
  Pmode : Inport
  Action Port : ActionPort  ActionPortLabel=else
  Pmode1 : Outport
  wires:
  Pmode/1 -> Pmode1/1

== system Shanthan_Heeirthan_EE469S3D_R45 (1)/control_law/CMD/CMDprocess/CommandTypes/Ramp2/Zcmd/Subsystem/Mode2 ==
  Pmode : Inport
  Action Port : ActionPort  ActionPortLabel=if(u1 ==0)
  Constant : Constant
  Sum : Sum  Inputs=|++
  Pmode1 : Outport
  wires:
  Pmode/1 -> Sum/1
  Constant/1 -> Sum/2
  Sum/1 -> Pmode1/1  "Pmode"

== system Shanthan_Heeirthan_EE469S3D_R45 (1)/control_law/CMD/CMDprocess/CommandTypes/Ramp2/Zcmd/Subsystem/Threshold ==
  Sensed : Inport
  CMDS : Inport  Port=2
  Abs : Abs  SaturateOnIntegerOverflow=off
  Bus to Vector : BusToVector
  Bus to Vector1 : BusToVector
  Constant1 : Constant  Value=[TOLdata(1,3);TOLdata(2,3)]
  Data Type Conversion : DataTypeConversion  OutDataTypeStr=double  SaturateOnIntegerOverflow=off  RndMeth=Floor
  Relational Operator : RelationalOperator  OutDataTypeStr=boolean  RndMeth=Simplest  InputSameDT=off
  Sum2 : Sum  Inputs=|+-
  Sum3 : Sum  Inputs=+
  Threshold : Outport
  wires:
  Sum2/1 -> Abs/1
  Bus to Vector/1 -> Sum2/1
  Bus to Vector1/1 -> Sum2/2
  Constant1/1 -> Relational Operator/2
  Abs/1 -> Relational Operator/1
  Data Type Conversion/1 -> Sum3/1
  Sensed/1 -> Bus to Vector1/1
  Relational Operator/1 -> Data Type Conversion/1
  CMDS/1 -> Bus to Vector/1
  Sum3/1 -> Threshold/1  "threshold"

== system Shanthan_Heeirthan_EE469S3D_R45 (1)/control_law/CMD/CMDprocess/CommandTypes/Ramp2/Zcmd/Subsystem/True ==
  Action Port : ActionPort  ActionPortLabel=if(u1 ==0)
  Constant : Constant
  Out1 : Outport
  wires:
  Constant/1 -> Out1/1  "one"

== system Shanthan_Heeirthan_EE469S3D_R45 (1)/control_law/CMD/CMDprocess/CommandTypes/Ramp3/Xcmd1/VariableTimer/DetectTFchange ==
  In1 : Inport
  In3 : Inport  Port=2
  Constant : Constant  Value=0
  Relational Operator1 : RelationalOperator  Operator=~=  OutDataTypeStr=boolean  RndMeth=Simplest  InputSameDT=off
  Switch3 : Switch  Criteria=u2 > Threshold  SaturateOnIntegerOverflow=off  InputSameDT=off
  Unit Delay : UnitDelay  InitialCondition=-dt  SampleTime=dt  HasFrameUpgradeWarning=on
  Out1 : Outport
  Out2 : Outport  Port=2
  wires:
  Switch3/1 -> Out1/1  "ResetValue"
  In3/1 -> Relational Operator1/1, Unit Delay/1
  Unit Delay/1 -> Relational Operator1/2
  Relational Operator1/1 -> Out2/1, Switch3/2  "Reset2"
  In1/1 -> Switch3/3
  Constant/1 -> Switch3/1

== system Shanthan_Heeirthan_EE469S3D_R45 (1)/control_law/CMD/CMDprocess/CommandTypes/Ramp3/Ycmd/VariableTimer/DetectTFchange ==
  In1 : Inport
  In3 : Inport  Port=2
  Constant : Constant  Value=0
  Relational Operator1 : RelationalOperator  Operator=~=  OutDataTypeStr=boolean  RndMeth=Simplest  InputSameDT=off
  Switch3 : Switch  Criteria=u2 > Threshold  SaturateOnIntegerOverflow=off  InputSameDT=off
  Unit Delay : UnitDelay  InitialCondition=-dt  SampleTime=dt  HasFrameUpgradeWarning=on
  Out1 : Outport
  Out2 : Outport  Port=2
  wires:
  Switch3/1 -> Out1/1  "ResetValue"
  In3/1 -> Relational Operator1/1, Unit Delay/1
  Unit Delay/1 -> Relational Operator1/2
  Relational Operator1/1 -> Out2/1, Switch3/2  "Reset2"
  In1/1 -> Switch3/3
  Constant/1 -> Switch3/1

== system Shanthan_Heeirthan_EE469S3D_R45 (1)/control_law/CMD/CMDprocess/CommandTypes/Ramp3/Zcmd/StartTimer/VariableTimer ==
  TFramp : Inport
  Constant : Constant  Value=dt
  DetectTFchange : Subsystem
  Logical Operator : Logic  Operator=OR  AllPortsSameDT=off  OutDataTypeStr=boolean
  Relational Operator : RelationalOperator  Operator=<=  OutDataTypeStr=boolean  RndMeth=Simplest  InputSameDT=off
  Sum : Sum  Inputs=|++
  Switch : Switch  Criteria=u2 > Threshold  SaturateOnIntegerOverflow=off  InputSameDT=off
  Unit Delay1 : UnitDelay  SampleTime=dt  HasFrameUpgradeWarning=on
  Unit Delay2 : UnitDelay  InitialCondition=-dt  SampleTime=dt  HasFrameUpgradeWarning=on
  Time_sec : Outport
  wires:
  Unit Delay2/1 -> Sum/2
  Sum/1 -> Relational Operator/2, Switch/3
  Constant/1 -> Sum/1
  Logical Operator/1 -> Switch/2
  Switch/1 -> Time_sec/1, Unit Delay1/1, Unit Delay2/1  "Time_sec"
  DetectTFchange/1(Out1) -> Switch/1
  Unit Delay1/1 -> DetectTFchange/1(In1)  "TimeZ_sec"
  DetectTFchange/2(Out2) -> Logical Operator/1
  TFramp/1 -> DetectTFchange/2(In3), Relational Operator/1
  Relational Operator/1 -> Logical Operator/2  "Reset1"

== system Shanthan_Heeirthan_EE469S3D_R45 (1)/control_law/CMD/CMDprocess/CommandTypes/Ramp3/Zcmd/Subsystem/False ==
  Action Port : ActionPort  ActionPortLabel=else
  Constant : Constant  Value=0
  Out1 : Outport
  wires:
  Constant/1 -> Out1/1  "zero"

== system Shanthan_Heeirthan_EE469S3D_R45 (1)/control_law/CMD/CMDprocess/CommandTypes/Ramp3/Zcmd/Subsystem/Mode1 ==
  Pmode : Inport
  Action Port : ActionPort  ActionPortLabel=else
  Pmode1 : Outport
  wires:
  Pmode/1 -> Pmode1/1

== system Shanthan_Heeirthan_EE469S3D_R45 (1)/control_law/CMD/CMDprocess/CommandTypes/Ramp3/Zcmd/Subsystem/Mode2 ==
  Pmode : Inport
  Action Port : ActionPort  ActionPortLabel=if(u1 ==0)
  Constant : Constant
  Sum : Sum  Inputs=|++
  Pmode1 : Outport
  wires:
  Pmode/1 -> Sum/1
  Constant/1 -> Sum/2
  Sum/1 -> Pmode1/1  "Pmode"

== system Shanthan_Heeirthan_EE469S3D_R45 (1)/control_law/CMD/CMDprocess/CommandTypes/Ramp3/Zcmd/Subsystem/Threshold ==
  Sensed : Inport
  CMDS : Inport  Port=2
  Abs : Abs  SaturateOnIntegerOverflow=off
  Bus to Vector : BusToVector
  Bus to Vector1 : BusToVector
  Constant1 : Constant  Value=[TOLdata(1,4);TOLdata(2,4)]
  Data Type Conversion : DataTypeConversion  OutDataTypeStr=double  SaturateOnIntegerOverflow=off  RndMeth=Floor
  Relational Operator : RelationalOperator  OutDataTypeStr=boolean  RndMeth=Simplest  InputSameDT=off
  Sum2 : Sum  Inputs=|+-
  Sum3 : Sum  Inputs=+
  Threshold : Outport
  wires:
  Sum2/1 -> Abs/1
  Bus to Vector/1 -> Sum2/1
  Bus to Vector1/1 -> Sum2/2
  Constant1/1 -> Relational Operator/2
  Abs/1 -> Relational Operator/1
  Data Type Conversion/1 -> Sum3/1
  Sensed/1 -> Bus to Vector1/1
  Relational Operator/1 -> Data Type Conversion/1
  CMDS/1 -> Bus to Vector/1
  Sum3/1 -> Threshold/1  "threshold"

== system Shanthan_Heeirthan_EE469S3D_R45 (1)/control_law/CMD/CMDprocess/CommandTypes/Ramp3/Zcmd/Subsystem/True ==
  Action Port : ActionPort  ActionPortLabel=if(u1 ==0)
  Constant : Constant
  Out1 : Outport
  wires:
  Constant/1 -> Out1/1  "one"

== system Shanthan_Heeirthan_EE469S3D_R45 (1)/control_law/CMD/CMDprocess/CommandTypes/Ramp4/Xcmd1/VariableTimer/DetectTFchange ==
  In1 : Inport
  In3 : Inport  Port=2
  Constant : Constant  Value=0
  Relational Operator1 : RelationalOperator  Operator=~=  OutDataTypeStr=boolean  RndMeth=Simplest  InputSameDT=off
  Switch3 : Switch  Criteria=u2 > Threshold  SaturateOnIntegerOverflow=off  InputSameDT=off
  Unit Delay : UnitDelay  InitialCondition=-dt  SampleTime=dt  HasFrameUpgradeWarning=on
  Out1 : Outport
  Out2 : Outport  Port=2
  wires:
  Switch3/1 -> Out1/1  "ResetValue"
  In3/1 -> Relational Operator1/1, Unit Delay/1
  Unit Delay/1 -> Relational Operator1/2
  Relational Operator1/1 -> Out2/1, Switch3/2  "Reset2"
  In1/1 -> Switch3/3
  Constant/1 -> Switch3/1

== system Shanthan_Heeirthan_EE469S3D_R45 (1)/control_law/CMD/CMDprocess/CommandTypes/Ramp4/Ycmd/VariableTimer/DetectTFchange ==
  In1 : Inport
  In3 : Inport  Port=2
  Constant : Constant  Value=0
  Relational Operator1 : RelationalOperator  Operator=~=  OutDataTypeStr=boolean  RndMeth=Simplest  InputSameDT=off
  Switch3 : Switch  Criteria=u2 > Threshold  SaturateOnIntegerOverflow=off  InputSameDT=off
  Unit Delay : UnitDelay  InitialCondition=-dt  SampleTime=dt  HasFrameUpgradeWarning=on
  Out1 : Outport
  Out2 : Outport  Port=2
  wires:
  Switch3/1 -> Out1/1  "ResetValue"
  In3/1 -> Relational Operator1/1, Unit Delay/1
  Unit Delay/1 -> Relational Operator1/2
  Relational Operator1/1 -> Out2/1, Switch3/2  "Reset2"
  In1/1 -> Switch3/3
  Constant/1 -> Switch3/1
